simulink subsystem "Navigation_Controller"  (R2023b)
settings: Solver=VariableStepAuto  StartTime=0.0  StopTime=10.0  RelTol=1e-3
undefined symbols (not defined in the file): KD_Lateral, KI_BCL, KP_BCL, KP_Lateral, KP_TECL
libraries: simulink_extras x3, slpidlib x2
settings Model: Creator=cyber  LastModifiedBy=cyber

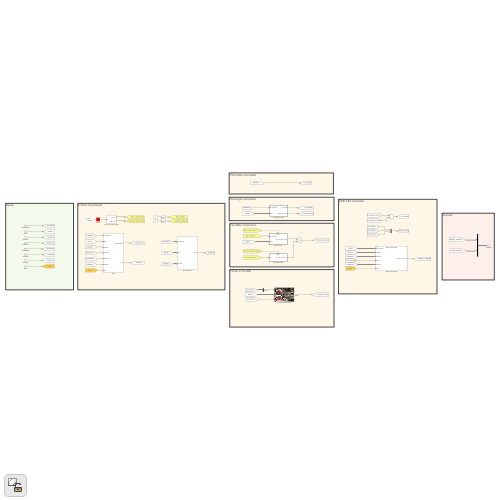
[thumbnail: Simulink's stored preview of the top-level diagram]
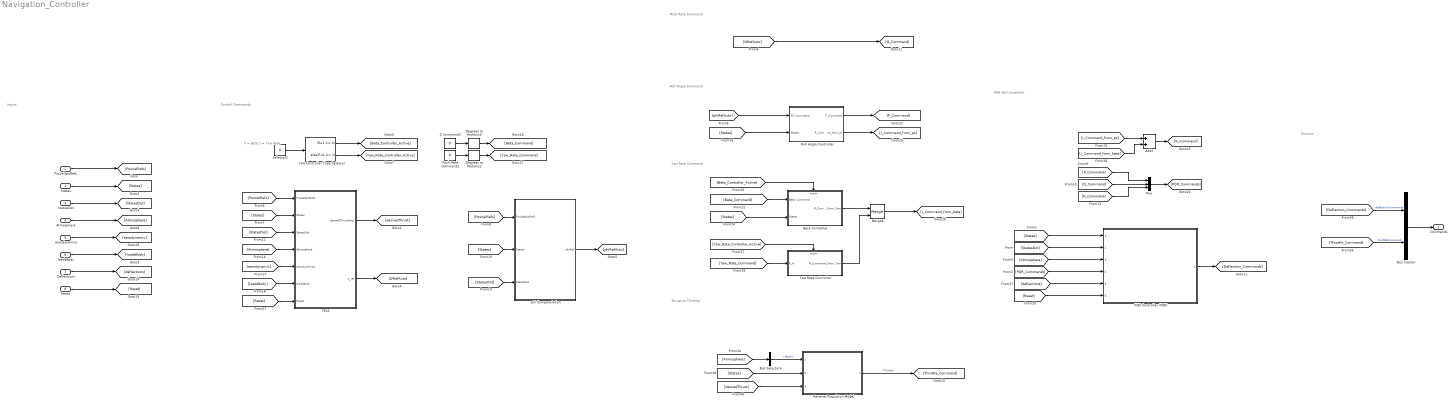
== system Navigation_Controller ==
  note: Pitch Rate Command
  note: 0 = Beta
      | 1 = Yaw Rate
  note: Control Commands
  note: Outputs
  note: Roll Angle Command
  note: Yaw Rate Command
  note: Thrust to Throttle
  note: PQR INDI Controller
  note: Inputs
  PosVelAccRefs : Inport
  States : Inport  Port=2
  StatesDot : Inport  Port=3
  Atmosphere : Inport  Port=4
  aerodynamics : Inport  Port=5
  loadsBody : Inport  Port=6
  Deflections : Inport  Port=7
  Reset : Inport  Port=8
  Add2 : Sum
  Beta Controller : Subsystem  TreatAsAtomicUnit=on
  Bus Creator : BusCreator  Inputs=2
  Bus Selector4 : BusSelector  OutputSignals=Mach
  Degrees to Radians2 : simulink_extras/Transformations/Degrees to Radians
  Degrees to Radians3 : simulink_extras/Transformations/Degrees to Radians
  G Command2 : Constant  Value=0
  INDI Controller (PQR) : Subsystem  ReferencedSubsystem=INDI_Controller_PQR
  Merge4 : Merge
  Mux : Mux  Inputs=3
  Pitch Rate Command2 : Constant  Value=0
  Reverse Propulsion Model : Subsystem  ReferencedSubsystem=Reverse_Propulsion_Model
  Roll Angle Controller : Subsystem  TreatAsAtomicUnit=on
  Selector2 : Constant  Value=0
      settings: OpenFcn=|
      | val = get_param(gcb,'Value')
      | 
      | switch val
      | case '1'
      | set_param(gcb,'Value','0')
      | set_param(gcb,'BackGroundColor','red')
      | otherwise
      | set_param(gcb,'Value','1')
      | set_param(gcb,'BackGroundColor','green')
      | end
  TECS : Subsystem
  Yaw Controller Type Selector : If  IfExpression=u1 == 0  ElseIfExpressions=u1 == 1  ShowElse=off
  Yaw Rate Controller : Subsystem
  phi Compansiation : Subsystem
  Commands : Outport
  wires:
  INDI Controller (PQR)/1 -> [Deflection_Commands]
  [States] -> INDI Controller (PQR)/1
  [Beta_Controller_Active] -> Beta Controller/Action
  phi Compansiation/1(phiRef) -> [phiRefAuto]
  [PosVelRefs] -> phi Compansiation/1(PosVelAccRefs)
  [Reset] -> INDI Controller (PQR)/6
  Bus Creator/1 -> Commands/1
  TECS/1(desiredThrustAuto) -> [desiredThrust]
  Reverse Propulsion Model/1 -> [Throttle_Command]  "Throttle"
  [PQR_Commands] -> INDI Controller (PQR)/4
  G Command2/1 -> Degrees to Radians3/1
  Degrees to Radians3/1 -> [Beta_Command]
  [Atmosphere] -> Bus Selector4/1
  Roll Angle Controller/1(P_Command) -> [P_Command]
  [StatesDot] -> INDI Controller (PQR)/2
  [phiRefAuto] -> Roll Angle Controller/1(Phi Command)
  [P_Command] -> Mux/1
  Add2/1 -> [R_Command]
  Yaw Controller Type Selector/2 -> [Yaw_Rate_Controller_Active]
  [desiredThrust] -> Reverse Propulsion Model/3
  TECS/2(q_ref) -> [QRefAuto]
  [States] -> Reverse Propulsion Model/2
  [QRefAuto] -> [Q_Command]
  [StatesDot] -> phi Compansiation/3(StatesDot)
  [States] -> phi Compansiation/2(States)
  [Yaw_Rate_Controller_Active] -> Yaw Rate Controller/Action
  Bus Selector4/1 -> Reverse Propulsion Model/1  "<Mach>"
  Mux/1 -> [PQR_Commands]
  [Deflection_Commands] -> Bus Creator/1  "deflectionCommands"
  [Beta_Command] -> Beta Controller/1(Beta Command)
  [Throttle_Command] -> Bus Creator/2  "throttleCommand"
  [r_Command_from_beta] -> Add2/2
  [r_Command_from_ps] -> Add2/1
  Yaw Controller Type Selector/1 -> [Beta_Controller_Active]
  Merge4/1 -> [r_Command_from_beta]
  [Q_Command] -> Mux/2
  Pitch Rate Command2/1 -> Degrees to Radians2/1
  [deflections] -> INDI Controller (PQR)/5
  Degrees to Radians2/1 -> [Yaw_Rate_Command]
  [Atmosphere] -> INDI Controller (PQR)/3
  [R_Command] -> Mux/3
  [States] -> Roll Angle Controller/2(States)
  Roll Angle Controller/2(R_Command_from_ps) -> [r_Command_from_ps]
  Yaw Rate Controller/1(R_Command_from_Yaw) -> Merge4/2
  [States] -> Beta Controller/2(States)
  Selector2/1 -> Yaw Controller Type Selector/1
  [Yaw_Rate_Command] -> Yaw Rate Controller/1(P_In)
  Beta Controller/1(R_Command_from_Yaw) -> Merge4/1
  PosVelAccRefs/1 -> [PosVelRefs]
  States/1 -> [States]
  StatesDot/1 -> [StatesDot]
  Atmosphere/1 -> [Atmosphere]
  aerodynamics/1 -> [aerodynamic]
  Reset/1 -> [Reset]
  Deflections/1 -> [deflections]
  loadsBody/1 -> [loadsBody]
  [PosVelRefs] -> TECS/1(PosVelAccRefs)
  [States] -> TECS/2(States)
  [StatesDot] -> TECS/3(StatesDot)
  [Atmosphere] -> TECS/4(Atmosphere)
  [aerodynamic] -> TECS/5(aerodynamics)
  [loadsBody] -> TECS/6(loadsBody)
  [Reset] -> TECS/7(Reset)

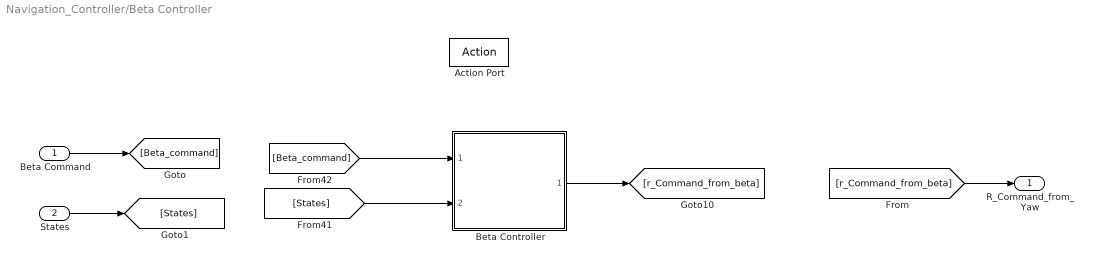
== system Navigation_Controller/Beta Controller ==
  Beta Command : Inport
  States : Inport  Port=2
  Action Port : ActionPort
  Beta Controller : Subsystem  ReferencedSubsystem=Beta_Controller
  R_Command_from_Yaw : Outport
  wires:
  Beta Controller/1 -> [r_Command_from_beta]
  [States] -> Beta Controller/2
  [Beta_command] -> Beta Controller/1
  Beta Command/1 -> [Beta_command]
  [r_Command_from_beta] -> R_Command_from_Yaw/1
  States/1 -> [States]

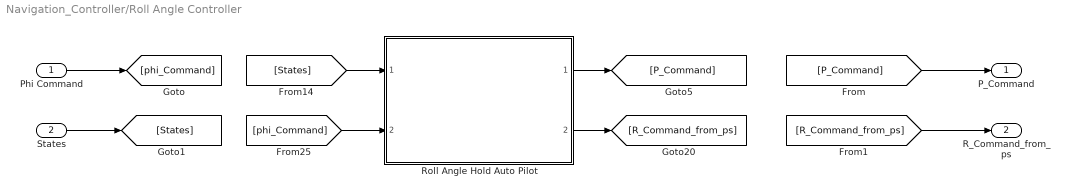
== system Navigation_Controller/Roll Angle Controller ==
  Phi Command : Inport
  States : Inport  Port=2
  "Roll Angle Hold Auto Pilot " : Subsystem  ReferencedSubsystem=Roll_Angle_Hold_Auto_Pilot
  P_Command : Outport
  R_Command_from_ps : Outport  Port=2
  wires:
  States/1 -> [States]
  [R_Command_from_ps] -> R_Command_from_ps/1
  [P_Command] -> P_Command/1
  Phi Command/1 -> [phi_Command]
  [States] -> "Roll Angle Hold Auto Pilot "/1
  [phi_Command] -> "Roll Angle Hold Auto Pilot "/2
  "Roll Angle Hold Auto Pilot "/1 -> [P_Command]
  "Roll Angle Hold Auto Pilot "/2 -> [R_Command_from_ps]

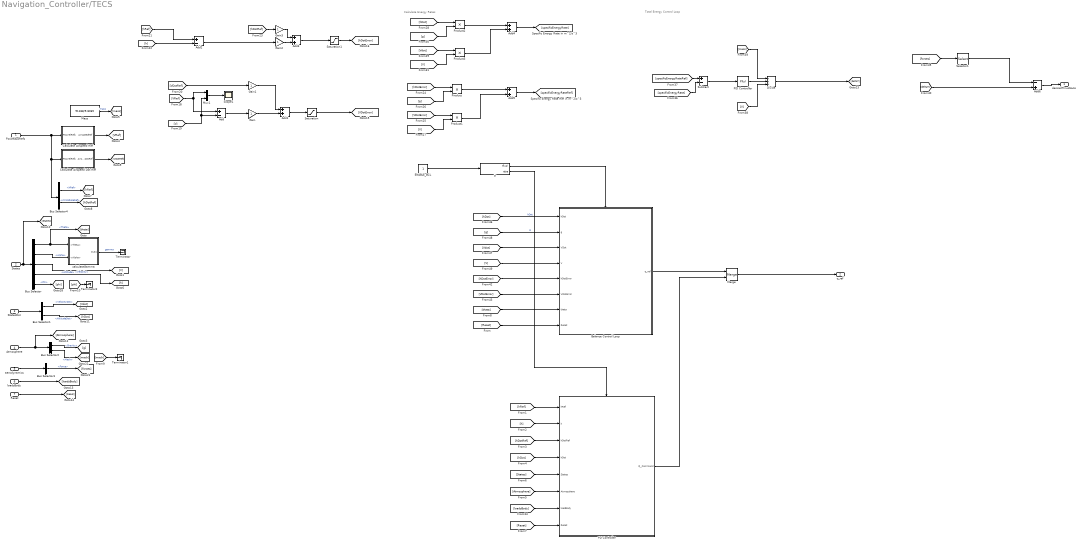
== system Navigation_Controller/TECS ==
  note: Calculate Energy Rates
  note: Total Energy Control Loop
  PosVelAccRefs : Inport
  States : Inport  Port=2
  StatesDot : Inport  Port=3
  Atmosphere : Inport  Port=4
  aerodynamics : Inport  Port=5
  loadsBody : Inport  Port=6
  Reset : Inport  Port=7
  Add : Sum  Inputs=+-
  Add{1,3..5} (4 alike) : Sum
  Add2 : Sum  Inputs=+-
  Add6 : Sum  Inputs=-+
  Balance Control Loop : Subsystem
  Bus Selector : BusSelector  OutputSignals=Theta,Alpha,Velocity,Altitude,Phi
  Bus Selector1 : BusSelector  OutputSignals=VelocityDot,AltitudeDot
  Bus Selector2 : BusSelector  OutputSignals=Gravity,Mach
  Bus Selector3 : BusSelector  OutputSignals=Force
  Bus Selector4 : BusSelector  OutputSignals=hRef,climbRateRef
  Calculate Airspeed Dot Ref : Subsystem
  Calculate Airspeed Ref : Subsystem
  Divide : Product  Inputs=**/
  ENABLE_BCL : Constant
      settings: OpenFcn=|
      | val = get_param(gcb,'Value')
      | 
      | switch val
      | case '1'
      | set_param(gcb,'Value','0')
      | set_param(gcb,'BackGroundColor','red')
      | otherwise
      | set_param(gcb,'Value','1')
      | set_param(gcb,'BackGroundColor','green')
      | end
  Gain{,1..3} (4 alike) : Gain
  If : If  IfExpression=u1
  Mass : Constant  Value=91188/9.8065
  Merge : Merge
  Mux1 : Mux  Inputs=2
  PD Controller : Subsystem
  PID Controller : slpidlib/PID Controller  Controller=PI  Form=Parallel  TimeDomain=Continuous-time  UseExternalTs=off  SampleTime=-1  IntegratorMethod=Forward Euler  FilterMethod=Forward Euler  ControllerParametersSource=internal  P=KP_TECL  I=0  UseKiTs=off  D=0  N=100  UseFilter=on  TunerSelectOption=Transfer Function Based (PID Tuner App)  InitialConditionSource=internal  InitialConditionForIntegrator=0  InitialConditionForFilter=0  DifferentiatorICPrevScaledInput=0  ExternalReset=none  TrackingMode=off  Kt=1  LimitOutput=off  SatLimitsSource=internal  UpperSaturationLimit=inf  LowerSaturationLimit=-inf  LinearizeAsGain=on  AntiWindupMode=none  Kb=1  LimitIntegrator=off  UpperIntegratorSaturationLimit=inf  LowerIntegratorSaturationLimit=-inf  POutMin=[]  POutMax=[]  IOutMin=[]  IOutMax=[]  DOutMin=[]  DOutMax=[]  NOutMin=[]  NOutMax=[]  SumOutMin=[]  SumOutMax=[]  SaturationOutMin=[]  SaturationOutMax=[]  PParamMin=[]  PParamMax=[]  IParamMin=[]  IParamMax=[]  DParamMin=[]  DParamMax=[]  NParamMin=[]  NParamMax=[]  KbParamMin=[]  KbParamMax=[]  KtParamMin=[]  KtParamMax=[]  KbOutMin=[]  KbOutMax=[]  KtOutMin=[]  KtOutMax=[]  IntegratorOutMin=[]  IntegratorOutMax=[]  FilterOutMin=[]  FilterOutMax=[]  SumI1OutMin=[]  SumI1OutMax=[]  SumI2OutMin=[]  SumI2OutMax=[]  SumI3OutMin=[]  SumI3OutMax=[]  SumI4OutMin=[]  SumI4OutMax=[]  SumDOutMin=[]  SumDOutMax=[]  DifferentiatorOutMin=[]  DifferentiatorOutMax=[]  FilterDiffOutCoefMin=[]  FilterDiffOutCoefMax=[]  ReciprocalOutMin=[]  ReciprocalOutMax=[]  SumDenOutMin=[]  SumDenOutMax=[]  SumNumOutMin=[]  SumNumOutMax=[]  DivideOutMin=[]  DivideOutMax=[]  UdiffTsProdOutMin=[]  UdiffTsProdOutMax=[]  NTsProdOutMin=[]  NTsProdOutMax=[]  UintegralTsProdOutMin=[]  UintegralTsProdOutMax=[]  UngainTsProdOutMin=[]  UngainTsProdOutMax=[]  ClampingZeroOutDataTypeStr=Inherit: Inherit via back propagation  ClampingZeroOutMin=[]  ClampingZeroOutMax=[]  FilterDenConstantOutDataTypeStr=Inherit: Inherit via back propagation  FilterDenConstantOutMin=[]  FilterDenConstantOutMax=[]  PCopyOutDataTypeStr=Inherit: Inherit via back propagation  PCopyOutMin=[]  PCopyOutMax=[]  NCopyOutDataTypeStr=Inherit: Inherit via back propagation  NCopyOutMin=[]  NCopyOutMax=[]  IntegratorContinuousStateAttributes=''  IntegratorStateMustResolveToSignalObject=off  IntegratorRTWStateStorageClass=Auto  FilterContinuousStateAttributes=''  FilterStateMustResolveToSignalObject=off  FilterRTWStateStorageClass=Auto  ParallelPVariant=InternalParameters  IdealPVariant=Disabled  IVariant=InternalParameters  DVariant=Disabled  IntegratorVariant=Continuous  SatVariant=Disabled  AWVariant=Passthrough  PCopyVariant=Disabled  TRVariant=Disabled  FdbkBlocksVariant=Forward  IdealPFdbkVariant=Disabled  SatFdbkVariant=Disabled  DerivativeFilterVariant=Disabled  NVariant=Disabled  NCopyVariant=Disabled_SignalSpec  FilterICVariant=Disabled  IntegratorICVariant=InternalICs  ExternalResetVariant=Disabled  TRSumVariant=Passthrough  SumFdbkVariant=Disabled  SumVariant=Sum_PI  TsampFilterVariant=InternalTs  TsampNgainVariant=Passthrough  TsampIntegralVariant=Disabled_SignalSpec  ExternalSaturationOutDataTypeStr=Inherit: Same as second input
  Product{,1..3} (4 alike) : Product
  Saturation : Saturate  UpperLimit=10  LowerLimit=-10
  Saturation1 : Saturate  UpperLimit=20  LowerLimit=-20
  Scope1 : Scope
  Selector1 : Selector  InputPortWidth=3  IndexOptions=Index vector (dialog)  Indices=1  OutputSizes=1
  Subtract : Sum  Inputs=+-
  Terminator : Terminator
  Terminator1 : Terminator
  Terminator2 : Terminator
  calculateGamma : Subsystem
  desiredThrustAuto : Outport
  q_ref : Outport  Port=2
  wires:
  Reset/1 -> [Reset]
  [phi] -> Terminator2/1
  [mach] -> Terminator1/1
  [theta] -> Balance Control Loop/7(theta)
  [Reset] -> PD Controller/8(Reset)
  [Reset] -> Balance Control Loop/8(Reset)
  loadsBody/1 -> [loadsBody]
  PD Controller/1(Q_Command) -> Merge/2
  [loadsBody] -> PD Controller/7(loadBody)
  [Atmosphere] -> PD Controller/6(Atmosphere)
  [States] -> PD Controller/5(States)
  [hDot] -> PD Controller/4(hDot)
  [hDotRef] -> PD Controller/3(hDotRef)
  [h] -> PD Controller/2(h)
  [hRef] -> PD Controller/1(hRef)
  If/2 -> PD Controller/Action
  Merge/1 -> q_ref/1
  If/1 -> Balance Control Loop/Action
  ENABLE_BCL/1 -> If/1
  Balance Control Loop/1(q_ref) -> Merge/1
  [VDotError] -> Balance Control Loop/6(VDotError)
  [hDotError] -> Balance Control Loop/5(hDotError)
  [V] -> Balance Control Loop/4(V)
  [Vdot] -> Balance Control Loop/3(VDot)
  [g] -> Balance Control Loop/2(g)  "g"
  [hDot] -> Balance Control Loop/1(hDot)  "hDot"
  Calculate Airspeed Dot Ref/1(AirspeedDotRef) -> [VDotRef]
  PosVelAccRefs/1 -> Calculate Airspeed Ref/1(PosVelRefs), Bus Selector4/1, Calculate Airspeed Dot Ref/1(PosVelRefs)
  Bus Selector4/2 -> [hDotRef]  "<climbRateRef>"
  Bus Selector4/1 -> [hRef]  "<hRef>"
  Calculate Airspeed Ref/1(AirspeedRef) -> [VRef]
  [VRef] -> Add/1, Mux1/1
  [V] -> Mux1/2, Add/2
  Mux1/1 -> Scope1/1
  Subtract/1 -> PID Controller/1
  Divide/1 -> [deltaT]
  PID Controller/1 -> Divide/2
  Bus Selector/5 -> [phi]  "<Phi>"
  Add6/1 -> desiredThrustAuto/1
  Selector1/1 -> Add6/1
  [deltaT] -> Add6/2
  [mass] -> Divide/1
  [V] -> Divide/3
  [specificEnergyRate] -> Subtract/2
  [specificEnergyRateRef] -> Subtract/1
  Bus Selector2/2 -> [mach]  "<Mach>"
  [forces] -> Selector1/1
  Bus Selector3/1 -> [forces]  "<Force>"
  aerodynamics/1 -> Bus Selector3/1
  Add5/1 -> [specificEnergyRateRef]
  Add4/1 -> [specificEnergyRate]
  [hDot] -> Product2/1
  [g] -> Product2/2
  Product2/1 -> Add4/1
  [Vdot] -> Product3/1
  [V] -> Product3/2
  Product3/1 -> Add4/2
  Product1/1 -> Add5/2
  [V] -> Product1/2
  [VDotError] -> Product1/1
  Product/1 -> Add5/1
  [g] -> Product/2
  [hDotError] -> Product/1
  Saturation1/1 -> [hDotError]
  Add3/1 -> Saturation1/1
  Gain3/1 -> Add3/1
  [hDotRef] -> Gain3/1
  Gain2/1 -> Add3/2
  Add2/1 -> Gain2/1
  [h] -> Add2/2
  Saturation/1 -> [VDotError]
  [hRef] -> Add2/1
  Add1/1 -> Saturation/1
  Gain1/1 -> Add1/1
  [VDotRef] -> Gain1/1
  Gain/1 -> Add1/2
  Add/1 -> Gain/1
  Bus Selector1/2 -> [hDot]  "<AltitudeDot>"
  Bus Selector/4 -> [h]  "<Altitude>"
  Mass/1 -> [mass]  "mass"
  Bus Selector2/1 -> [g]  "<Gravity>"
  Atmosphere/1 -> Bus Selector2/1, [Atmosphere]
  Bus Selector1/1 -> [Vdot]  "<VelocityDot>"
  StatesDot/1 -> Bus Selector1/1
  Bus Selector/3 -> [V]  "<Velocity>"
  calculateGamma/1(Out1) -> Terminator/1  "gamma"
  States/1 -> Bus Selector/1, [States]
  Bus Selector/1 -> calculateGamma/1(<Theta>), [theta]  "<Theta>"
  Bus Selector/2 -> calculateGamma/2(<Alpha>)  "<Alpha>"

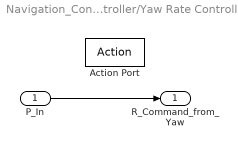
== system Navigation_Controller/Yaw Rate Controller ==
  P_In : Inport
  Action Port : ActionPort
  R_Command_from_Yaw : Outport
  wires:
  P_In/1 -> R_Command_from_Yaw/1

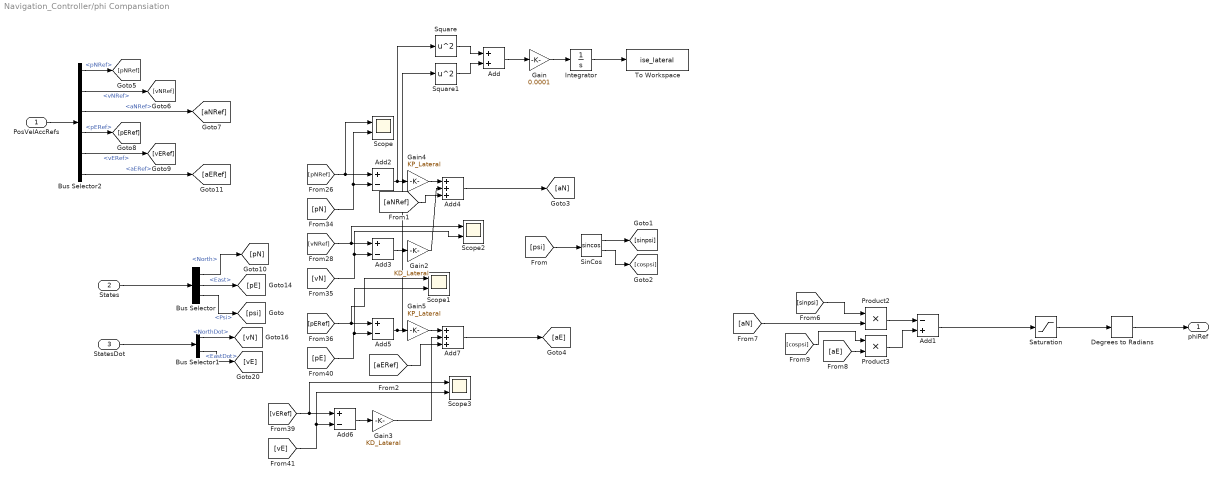
== system Navigation_Controller/phi Compansiation ==
  PosVelAccRefs : Inport
  States : Inport  Port=2
  StatesDot : Inport  Port=3
  Add : Sum
  Add1 : Sum  Inputs=-+
  Add{2..3,5..6} (4 alike) : Sum  Inputs=+-
  Add4 : Sum  Inputs=+++
  Add7 : Sum  Inputs=+++
  Bus Selector : BusSelector  OutputSignals=North,East,Psi
  Bus Selector1 : BusSelector  OutputSignals=NorthDot,EastDot
  Bus Selector2 : BusSelector  OutputSignals=pNRef,vNRef,aNRef,pERef,vERef,aERef
  Degrees to Radians : simulink_extras/Transformations/Degrees to Radians
  Gain : Gain  Gain=0.0001
  Gain2 : Gain  Gain=KD_Lateral
  Gain3 : Gain  Gain=KD_Lateral
  Gain4 : Gain  Gain=KP_Lateral
  Gain5 : Gain  Gain=KP_Lateral
  Integrator : Integrator
  Product2 : Product
  Product3 : Product
  Saturation : Saturate  UpperLimit=60  LowerLimit=-60
  Scope{,1..3} (4 alike) : Scope  NumInputPorts=2
  SinCos : Trigonometry  Operator=sincos
  Square : Math  Operator=square
  Square1 : Math  Operator=square
  To Workspace : ToWorkspace  VariableName=ise_lateral  SaveFormat=Timeseries  SampleTime=-1
  phiRef : Outport
  wires:
  [aERef] -> Add7/3
  [aNRef] -> Add4/3
  Bus Selector2/6 -> [aERef]  "<aERef>"
  Bus Selector2/5 -> [vERef]  "<vERef>"
  Bus Selector2/4 -> [pERef]  "<pERef>"
  Bus Selector2/3 -> [aNRef]  "<aNRef>"
  Bus Selector2/2 -> [vNRef]  "<vNRef>"
  Bus Selector2/1 -> [pNRef]  "<pNRef>"
  PosVelAccRefs/1 -> Bus Selector2/1
  Add1/1 -> Saturation/1
  Gain/1 -> Integrator/1
  Integrator/1 -> To Workspace/1
  Square1/1 -> Add/2
  Square/1 -> Add/1
  Add/1 -> Gain/1
  Gain5/1 -> Add7/1
  Gain4/1 -> Add4/1
  Degrees to Radians/1 -> phiRef/1
  [pERef] -> Add5/1, Scope1/1
  [pE] -> Add5/2, Scope1/2
  Gain3/1 -> Add7/2
  Gain2/1 -> Add4/2
  Add4/1 -> [aN]
  Saturation/1 -> Degrees to Radians/1
  [aN] -> Product2/2
  [sinpsi] -> Product2/1
  [aE] -> Product3/2
  Product2/1 -> Add1/1
  [cospsi] -> Product3/1
  Product3/1 -> Add1/2
  SinCos/2 -> [cospsi]
  SinCos/1 -> [sinpsi]
  [psi] -> SinCos/1
  Bus Selector/3 -> [psi]  "<Psi>"
  StatesDot/1 -> Bus Selector1/1
  States/1 -> Bus Selector/1
  Bus Selector/1 -> [pN]  "<North>"
  Add5/1 -> Gain5/1, Square1/1
  [vERef] -> Add6/1, Scope3/1
  [vE] -> Add6/2, Scope3/2
  Bus Selector1/1 -> [vN]  "<NorthDot>"
  [pNRef] -> Add2/1, Scope/1
  [vNRef] -> Add3/1, Scope2/1
  [pN] -> Add2/2, Scope/2
  Bus Selector/2 -> [pE]  "<East>"
  [vN] -> Add3/2, Scope2/2
  Add6/1 -> Gain3/1
  Add3/1 -> Gain2/1
  Add7/1 -> [aE]
  Bus Selector1/2 -> [vE]  "<EastDot>"
  Add2/1 -> Gain4/1, Square/1

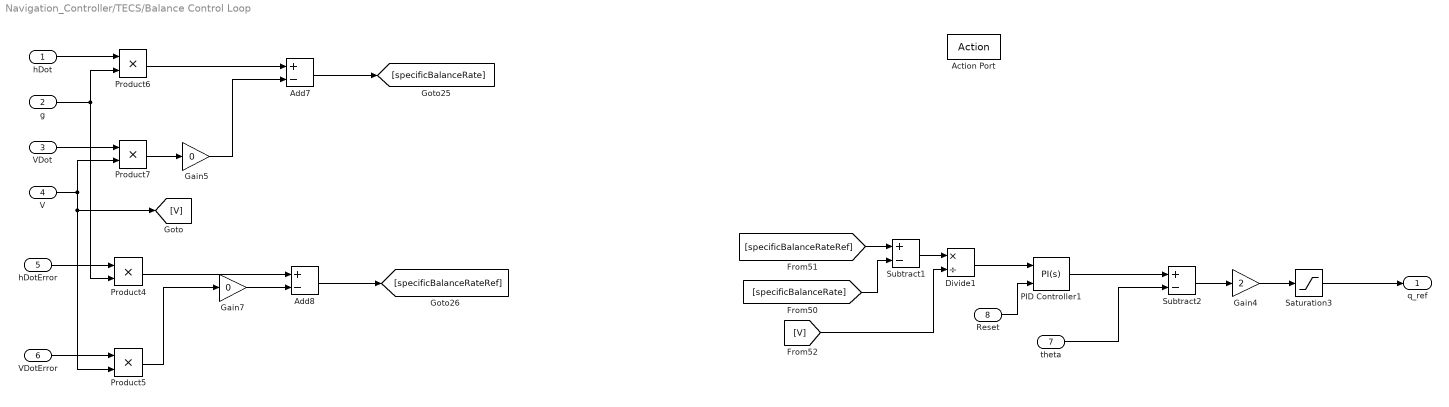
== system Navigation_Controller/TECS/Balance Control Loop ==
  hDot : Inport
  g : Inport  Port=2
  VDot : Inport  Port=3
  V : Inport  Port=4
  hDotError : Inport  Port=5
  VDotError : Inport  Port=6
  theta : Inport  Port=7
  Reset : Inport  Port=8
  Action Port : ActionPort
  Add7 : Sum  Inputs=+-
  Add8 : Sum  Inputs=+-
  Divide1 : Product  Inputs=*/
  Gain4 : Gain  Gain=2
  Gain5 : Gain  Gain=0
  Gain7 : Gain  Gain=0
  PID Controller1 : slpidlib/PID Controller  Controller=PI  Form=Parallel  TimeDomain=Continuous-time  UseExternalTs=off  SampleTime=-1  IntegratorMethod=Forward Euler  FilterMethod=Forward Euler  ControllerParametersSource=internal  P=KP_BCL  I=KI_BCL  UseKiTs=off  D=0  N=100  UseFilter=on  TunerSelectOption=Transfer Function Based (PID Tuner App)  InitialConditionSource=internal  InitialConditionForIntegrator=0  InitialConditionForFilter=0  DifferentiatorICPrevScaledInput=0  ExternalReset=either  TrackingMode=off  Kt=1  LimitOutput=off  SatLimitsSource=internal  UpperSaturationLimit=inf  LowerSaturationLimit=-inf  LinearizeAsGain=on  AntiWindupMode=none  Kb=1  LimitIntegrator=off  UpperIntegratorSaturationLimit=inf  LowerIntegratorSaturationLimit=-inf  POutMin=[]  POutMax=[]  IOutMin=[]  IOutMax=[]  DOutMin=[]  DOutMax=[]  NOutMin=[]  NOutMax=[]  SumOutMin=[]  SumOutMax=[]  SaturationOutMin=[]  SaturationOutMax=[]  PParamMin=[]  PParamMax=[]  IParamMin=[]  IParamMax=[]  DParamMin=[]  DParamMax=[]  NParamMin=[]  NParamMax=[]  KbParamMin=[]  KbParamMax=[]  KtParamMin=[]  KtParamMax=[]  KbOutMin=[]  KbOutMax=[]  KtOutMin=[]  KtOutMax=[]  IntegratorOutMin=[]  IntegratorOutMax=[]  FilterOutMin=[]  FilterOutMax=[]  SumI1OutMin=[]  SumI1OutMax=[]  SumI2OutMin=[]  SumI2OutMax=[]  SumI3OutMin=[]  SumI3OutMax=[]  SumI4OutMin=[]  SumI4OutMax=[]  SumDOutMin=[]  SumDOutMax=[]  DifferentiatorOutMin=[]  DifferentiatorOutMax=[]  FilterDiffOutCoefMin=[]  FilterDiffOutCoefMax=[]  ReciprocalOutMin=[]  ReciprocalOutMax=[]  SumDenOutMin=[]  SumDenOutMax=[]  SumNumOutMin=[]  SumNumOutMax=[]  DivideOutMin=[]  DivideOutMax=[]  UdiffTsProdOutMin=[]  UdiffTsProdOutMax=[]  NTsProdOutMin=[]  NTsProdOutMax=[]  UintegralTsProdOutMin=[]  UintegralTsProdOutMax=[]  UngainTsProdOutMin=[]  UngainTsProdOutMax=[]  ClampingZeroOutDataTypeStr=Inherit: Inherit via back propagation  ClampingZeroOutMin=[]  ClampingZeroOutMax=[]  FilterDenConstantOutDataTypeStr=Inherit: Inherit via back propagation  FilterDenConstantOutMin=[]  FilterDenConstantOutMax=[]  PCopyOutDataTypeStr=Inherit: Inherit via back propagation  PCopyOutMin=[]  PCopyOutMax=[]  NCopyOutDataTypeStr=Inherit: Inherit via back propagation  NCopyOutMin=[]  NCopyOutMax=[]  IntegratorContinuousStateAttributes=''  IntegratorStateMustResolveToSignalObject=off  IntegratorRTWStateStorageClass=Auto  FilterContinuousStateAttributes=''  FilterStateMustResolveToSignalObject=off  FilterRTWStateStorageClass=Auto  ParallelPVariant=InternalParameters  IdealPVariant=Disabled  IVariant=InternalParameters  DVariant=Disabled  IntegratorVariant=Continuous  SatVariant=Disabled  AWVariant=Passthrough  PCopyVariant=Disabled  TRVariant=Disabled  FdbkBlocksVariant=Forward  IdealPFdbkVariant=Disabled  SatFdbkVariant=Disabled  DerivativeFilterVariant=Disabled  NVariant=Disabled  NCopyVariant=Disabled_SignalSpec  FilterICVariant=Disabled  IntegratorICVariant=InternalICs  ExternalResetVariant=ExternalReset  TRSumVariant=Passthrough  SumFdbkVariant=Disabled  SumVariant=Sum_PI  TsampFilterVariant=InternalTs  TsampNgainVariant=Passthrough  TsampIntegralVariant=Disabled_SignalSpec  ExternalSaturationOutDataTypeStr=Inherit: Same as second input
  Product{4..7} (4 alike) : Product
  Saturation3 : Saturate  UpperLimit=20*pi/180  LowerLimit=-20*pi/180
  Subtract1 : Sum  Inputs=+-
  Subtract2 : Sum  Inputs=+-
  q_ref : Outport
  wires:
  Reset/1 -> PID Controller1/2
  VDot/1 -> Product7/1
  hDotError/1 -> Product4/1
  hDot/1 -> Product6/1
  [specificBalanceRate] -> Subtract1/2
  [V] -> Divide1/2
  Gain7/1 -> Add8/2
  theta/1 -> Subtract2/2
  g/1 -> Product4/2, Product6/2
  V/1 -> Product7/2, Product5/2, [V]
  Subtract2/1 -> Gain4/1
  Subtract1/1 -> Divide1/1
  Product6/1 -> Add7/1
  Product4/1 -> Add8/1
  PID Controller1/1 -> Subtract2/1
  Divide1/1 -> PID Controller1/1
  Product7/1 -> Gain5/1
  Saturation3/1 -> q_ref/1
  VDotError/1 -> Product5/1
  Add7/1 -> [specificBalanceRate]
  [specificBalanceRateRef] -> Subtract1/1
  Gain4/1 -> Saturation3/1
  Add8/1 -> [specificBalanceRateRef]
  Gain5/1 -> Add7/2
  Product5/1 -> Gain7/1

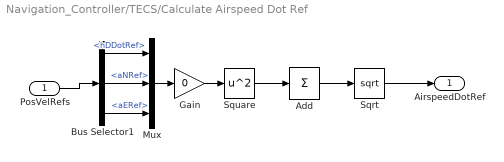
== system Navigation_Controller/TECS/Calculate Airspeed Dot Ref ==
  PosVelRefs : Inport
  Add : Sum  Inputs=+
  Bus Selector1 : BusSelector  OutputSignals=hDDotRef,aNRef,aERef
  Gain : Gain  Gain=0
  Mux : Mux  Inputs=3
  Sqrt : Sqrt
  Square : Math  Operator=square
  AirspeedDotRef : Outport
  wires:
  Gain/1 -> Square/1
  Bus Selector1/3 -> Mux/3  "<aERef>"
  Bus Selector1/2 -> Mux/2  "<aNRef>"
  Bus Selector1/1 -> Mux/1  "<hDDotRef>"
  Mux/1 -> Gain/1
  Sqrt/1 -> AirspeedDotRef/1
  Square/1 -> Add/1
  Add/1 -> Sqrt/1
  PosVelRefs/1 -> Bus Selector1/1

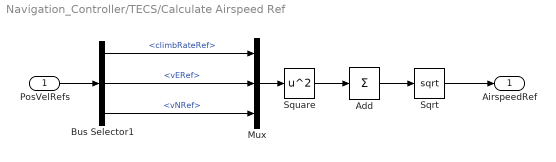
== system Navigation_Controller/TECS/Calculate Airspeed Ref ==
  PosVelRefs : Inport
  Add : Sum  Inputs=+
  Bus Selector1 : BusSelector  OutputSignals=climbRateRef,vERef,vNRef
  Mux : Mux  Inputs=3
  Sqrt : Sqrt
  Square : Math  Operator=square
  AirspeedRef : Outport
  wires:
  PosVelRefs/1 -> Bus Selector1/1
  Add/1 -> Sqrt/1
  Bus Selector1/1 -> Mux/1  "<climbRateRef>"
  Square/1 -> Add/1
  Sqrt/1 -> AirspeedRef/1
  Bus Selector1/2 -> Mux/2  "<vERef>"
  Mux/1 -> Square/1
  Bus Selector1/3 -> Mux/3  "<vNRef>"

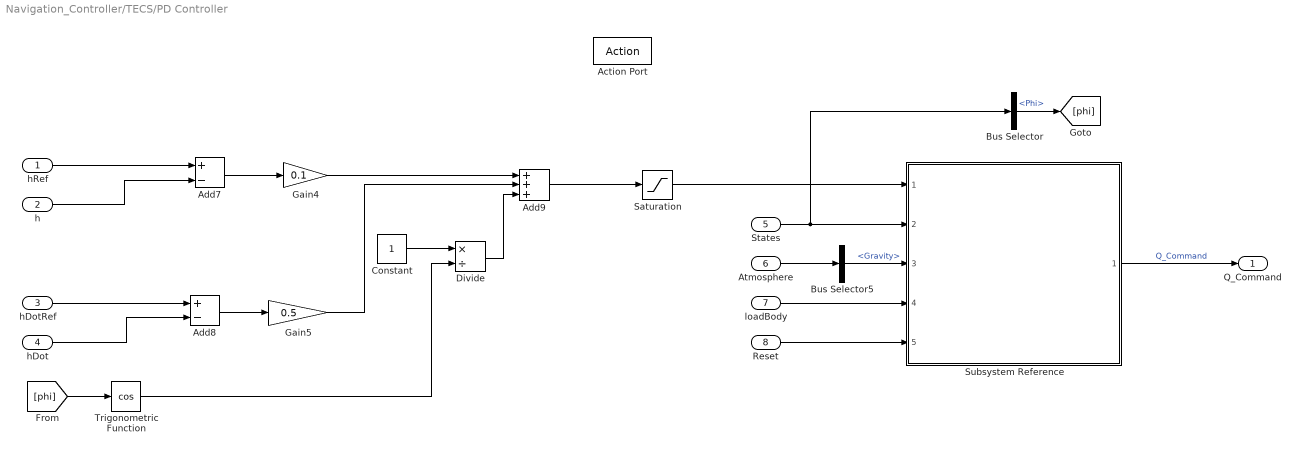
== system Navigation_Controller/TECS/PD Controller ==
  hRef : Inport
  h : Inport  Port=2
  hDotRef : Inport  Port=3
  hDot : Inport  Port=4
  States : Inport  Port=5
  Atmosphere : Inport  Port=6
  loadBody : Inport  Port=7
  Reset : Inport  Port=8
  Action Port : ActionPort
  Add7 : Sum  Inputs=+-
  Add8 : Sum  Inputs=+-
  Add9 : Sum  Inputs=+++
  Bus Selector : BusSelector  OutputSignals=Phi
  Bus Selector5 : BusSelector  OutputSignals=Gravity
  Constant : Constant
  Divide : Product  Inputs=*/
  Gain4 : Gain  Gain=0.1
  Gain5 : Gain  Gain=0.5
  Saturation : Saturate  UpperLimit=5  LowerLimit=-3
  Subsystem Reference : Subsystem  ReferencedSubsystem=G_Command_to_PQR_Command
  Trigonometric Function : Trigonometry  Operator=cos
  Q_Command : Outport
  wires:
  Divide/1 -> Add9/3
  Constant/1 -> Divide/1
  Trigonometric Function/1 -> Divide/2
  [phi] -> Trigonometric Function/1
  Bus Selector/1 -> [phi]  "<Phi>"
  Saturation/1 -> Subsystem Reference/1
  Reset/1 -> Subsystem Reference/5
  hRef/1 -> Add7/1
  h/1 -> Add7/2
  hDot/1 -> Add8/2
  Atmosphere/1 -> Bus Selector5/1
  loadBody/1 -> Subsystem Reference/4
  Add8/1 -> Gain5/1
  Gain5/1 -> Add9/2
  Subsystem Reference/1 -> Q_Command/1  "Q_Command"
  Bus Selector5/1 -> Subsystem Reference/3  "<Gravity>"
  Add9/1 -> Saturation/1
  States/1 -> Subsystem Reference/2, Bus Selector/1
  Add7/1 -> Gain4/1
  Gain4/1 -> Add9/1
  hDotRef/1 -> Add8/1

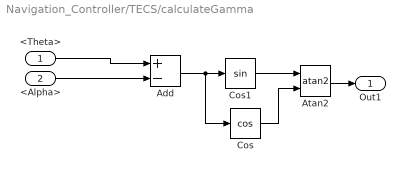
== system Navigation_Controller/TECS/calculateGamma ==
  <Theta> : Inport
  <Alpha> : Inport  Port=2
  Add : Sum  Inputs=+-
  Atan2 : Trigonometry  Operator=atan2
  Cos : Trigonometry  Operator=cos
  Cos1 : Trigonometry
  Out1 : Outport
  wires:
  Atan2/1 -> Out1/1
  <Alpha>/1 -> Add/2
  Add/1 -> Cos1/1, Cos/1
  <Theta>/1 -> Add/1
  Cos1/1 -> Atan2/1
  Cos/1 -> Atan2/2
